simulink model "Six_Step_Commutation"  (R2022b)
settings: Solver=FixedStepAuto  StartTime=0.0  StopTime=inf  FixedStep=50e-6  RelTol=1e-3
undefined symbols (not defined in the file): IO397, pull, up
libraries: speedgoatlib_fpga_pwm x1, speedgoatlib_fpga_dio x1, simulink x1, speedgoatlib_fpga x1
settings Model: SimulationMode=external  ExtModeEnableFloating=off  ExtModeTrigDuration=100000  Creator=safder.1  LastModifiedBy=safder.1
settings SolverCC: ConcurrentTasks=on  PositivePriorityOrder=on  AutoInsertRateTranBlk=on
settings OptimizationCC: BlockReduction=off  OptimizeBlockIOStorage=off
settings DebuggingCC: TasksWithSamePriorityMsg=none
settings HardwareCC: ProdBitPerLong=64  ProdLongLongMode=on  ProdHWDeviceType=Intel->x86-64 (Linux 64)
settings RTWCC: Description=Simulink Real-Time  SystemTargetFile=slrealtime.tlc  TemplateMakefile=slrealtime_default_tmf  Toolchain=Simulink Real-Time Toolchain  BuildConfiguration=Faster Runs  CodeExecutionProfiling=on  TargetLang=C++

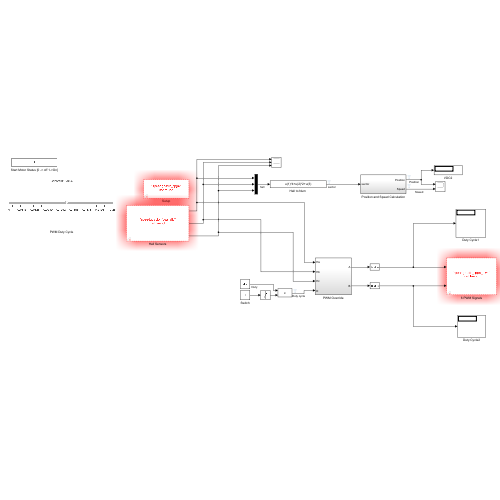
[thumbnail: Simulink's stored preview of the top-level diagram]
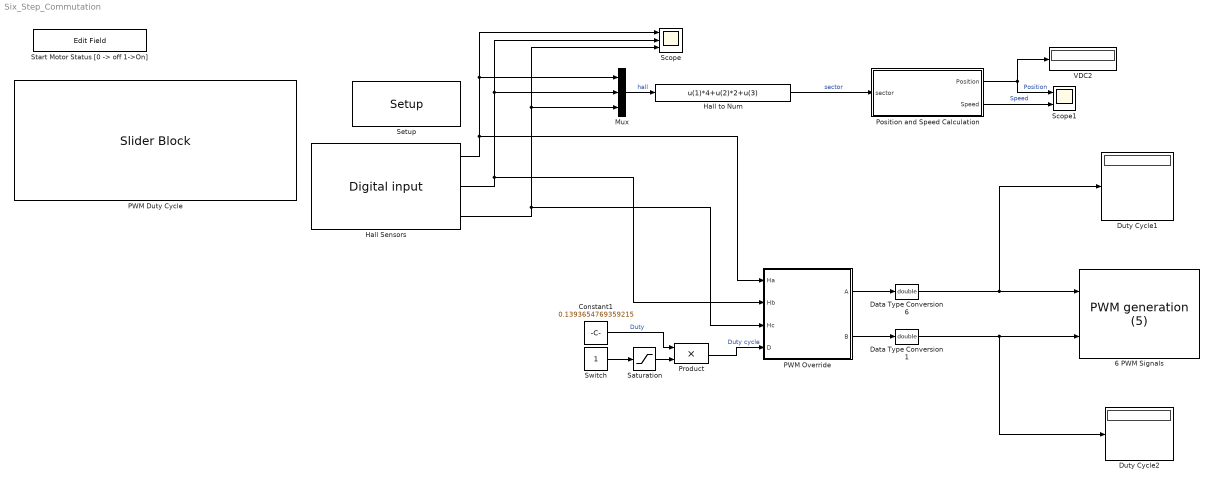
== system Six_Step_Commutation ==
  6 PWM Signals : speedgoatlib_fpga_pwm/PWM generation (5)  id=1  chan=[1 2 3]  board=Please select...  ts=0.0001  enableDma=off  pciSlot=-1  delay=0  symmetric=Symmetric - PWM generation is centered around half the period  b_is_complement_of_a=Independent of PWM A output  deadband=[0.0000025]  period=0.0001  frequency=10000  ticks=7499  a_on=[0]  a_off=[0]  pwm_a_dc=[0.0]  b_on=[0]  b_off=[0]  pwm_b_dc=[0]  c_on=[0.0]  c_off=[0.0]  protection=Disabled: A and B can be high at the same moment  enable_latch_half_period=off  pwm_update=At period starts  bit_width_pwm_gen=24  trigger_duration=[1e-6]  trigger_period_start=off  trigger_half_of_the_period=off  trigger_a_on=off  trigger_a_off=off  trigger_b_on=off  trigger_b_off=off  show_a_input=on  show_b_input=on  show_c_input=off  show_period_input=off  show_force_stop_input=off  idle_a=Low when PWM generation is halted  idle_b=Low when PWM generation is halted  idle_c=Low when PWM generation is halted  cancels_pwm_generation=on  invert_a=off  invert_b=off  invert_c=off
  Constant1 : Constant  Value=0.1393654769359215
  Data Type Conversion1 : DataTypeConversion  OutDataTypeStr=double  SaturateOnIntegerOverflow=off  RndMeth=Floor
  Data Type Conversion6 : DataTypeConversion  OutDataTypeStr=double  SaturateOnIntegerOverflow=off  RndMeth=Floor
  Duty Cycle1 : Display
  Duty Cycle2 : Display
  Hall Sensors : speedgoatlib_fpga_dio/Digital input  id=1  chan=[11 12 13]  ts=0.0001  vectorizeOutput=off
  "Hall to Num " : Fcn  Expr=u(1)*4+u(2)*2+u(3)
  Mux : Mux  Inputs=3
  PWM Duty Cycle : SliderBlock  ScaleMax=0.25
  PWM Override : Subsystem
  Position and Speed Calculation : Subsystem
  Product : Product
  Saturation : Saturate  UpperLimit=1  LowerLimit=0
  Scope : Scope  NumInputPorts=3
  Scope1 : Scope  NumInputPorts=2
  Setup : speedgoatlib_fpga/Setup/Setup  Parameter124={}  board=IO397-50k  id=1  pciSlot=-1  device_id=1  bitstreamFilePath=C:\ProgramData\Speedgoat\bitstreams\io_configuration_package\R2022b\io397  bitstreamFile=speedgoat_IO397_RCP.mat  rearEnb_1=off  rearIO_1=None  rearEnb_2=off  rearIO_2=None  ProgSpiFlash=off  ProgBPIFlash=off  useFpgaDmaController=off  PullRPort15=pull-up 3.3V  PullRPort31=pull-up 3.3V  PullRPort47=pull-up 3.3V  PullRPort63=pull-up 3.3V  diffLineTermination_1=on  diffLineTermination_2=on  diffLineTermination_3=on  diffLineTermination_4=on  diffLineTermination_5=on  diffLineTermination_6=on  diffLineTermination_7=on  diffLineTermination_8=on  diffLineTermination_9=on  diffLineTermination_10=on  diffLineTermination_11=on  diffLineTermination_12=on  diffLineTermination_13=on  diffLineTermination_14=on  diffLineTermination_15=on  diffLineTermination_16=on  diffLineTermination_17=on  diffLineTermination_18=on  diffLineTermination_19=on  diffLineTermination_20=on  diffLineTermination_21=on  diffLineTermination_22=on  diffLineTermination_23=on  diffLineTermination_24=on  diffLineTermination_25=on  diffLineTermination_26=on  diffLineTermination_27=on  diffLineTermination_28=on  diffLineTermination_29=on  diffLineTermination_30=on  diffLineTermination_31=on  diffLineTermination_32=on  Vi_Pull_36x_1=Floating  Vo_36x_1=3.3V  Vi_Pull_36x_2=Floating  Vo_36x_2=3.3V  Vi_Pull_36x_3=Floating  Vo_36x_3=3.3V  Vi_Pull_36x_4=Floating  Vo_36x_4=3.3V  Vi_Pull_36x_5=Floating  Vo_36x_5=3.3V  Vi_Pull_36x_6=Floating  Vo_36x_6=3.3V  Vi_Pull_36x_7=Floating  Vo_36x_7=3.3V  Vi_Pull_36x_8=Floating  Vo_36x_8=3.3V  Vi_Pull_36x_9_16=Floating  Vo_36x_9_16=3.3V  Vi_Pull_36x_17_24=Floating  Vo_36x_17_24=3.3V  Vi_Pull_36x_25_32=Floating  Vo_36x_25_32=3.3V  Vi_Pull_36x_33_40=Floating  Vo_36x_33_40=3.3V  Vi_Pull_36x_41_48=Floating  Vo_36x_41_48=3.3V  Vi_Pull_36x_49_56=Floating  Vo_36x_49_56=3.3V  Vi_Pull_36x_57_64=Floating  Vo_36x_57_64=3.3V  PullRPort0_1=pull-up  VioPort0_1=3.3V  PullRPort1_1=pull-up  VioPort1_1=3.3V  PullRPort2_1=pull-up  VioPort2_1=3.3V  PullRPort3_1=pull-up  VioPort3_1=3.3V  PullRPort4_1=pull-up  VioPort4_1=3.3V  PullRPort5_1=pull-up  VioPort5_1=3.3V  PullRPort6_1=pull-up  VioPort6_1=3.3V  diffLineTermination_rear1_1=on  diffLineTermination_rear1_2=on  diffLineTermination_rear1_3=on  diffLineTermination_rear1_4=on  diffLineTermination_rear1_5=on  diffLineTermination_rear1_6=on  diffLineTermination_rear1_7=on  diffLineTermination_rear1_8=on  PullRPort0_2=pull-up  VioPort0_2=3.3V  PullRPort1_2=pull-up  VioPort1_2=3.3V  PullRPort2_2=pull-up  VioPort2_2=3.3V  PullRPort3_2=pull-up  VioPort3_2=3.3V  PullRPort4_2=pull-up  VioPort4_2=3.3V  PullRPort5_2=pull-up  VioPort5_2=3.3V  PullRPort6_2=pull-up  VioPort6_2=3.3V  diffLineTermination_rear2_1=on  diffLineTermination_rear2_2=on  diffLineTermination_rear2_3=on  diffLineTermination_rear2_4=on  diffLineTermination_rear2_5=on  diffLineTermination_rear2_6=on  diffLineTermination_rear2_7=on  diffLineTermination_rear2_8=on
  "Start Motor Status [0 -> off 1->On]" : EditField  LabelPosition=Hide  ShowInitialText=on  Alignment=Center
  Switch : Constant
  VDC2 : Display
  wires:
  Mux/1 -> "Hall to Num "/1  "hall"
  Hall Sensors/1 -> PWM Override/1(Ha), Scope/1, Mux/1
  Hall Sensors/2 -> Mux/2, Scope/2, PWM Override/2(Hb)
  Hall Sensors/3 -> PWM Override/3(Hc), Scope/3, Mux/3
  PWM Override/1(A) -> Data Type Conversion6/1
  PWM Override/2(B) -> Data Type Conversion1/1
  Data Type Conversion6/1 -> 6 PWM Signals/1, Duty Cycle1/1
  Data Type Conversion1/1 -> 6 PWM Signals/2, Duty Cycle2/1
  "Hall to Num "/1 -> Position and Speed Calculation/1(sector)  "sector"
  Position and Speed Calculation/2(Speed) -> Scope1/2  "Speed"
  Position and Speed Calculation/1(Position) -> VDC2/1, Scope1/1  "Position"
  Switch/1 -> Saturation/1
  Saturation/1 -> Product/2
  Constant1/1 -> Product/1  "Duty"
  Product/1 -> PWM Override/4(D)  "Duty cycle"

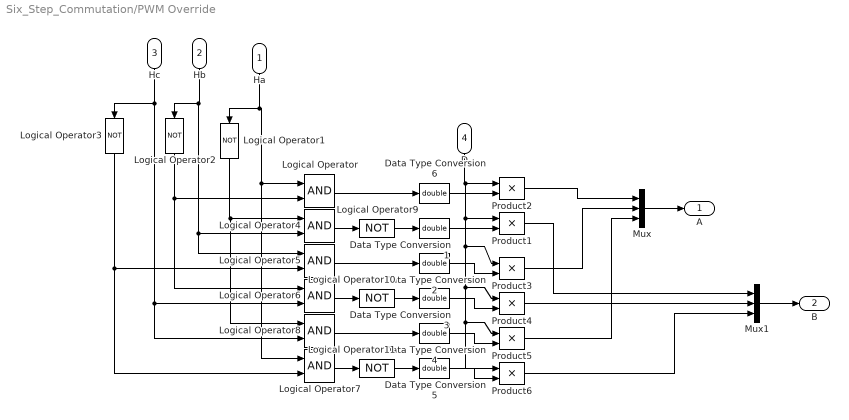
== system Six_Step_Commutation/PWM Override ==
  Ha : Inport
  Hb : Inport  Port=2
  Hc : Inport  Port=3
  D : Inport  Port=4
  Data Type Conversion{1..6} (6 alike) : DataTypeConversion  OutDataTypeStr=double  SaturateOnIntegerOverflow=off  RndMeth=Floor
  Logical Operator{,4..8} (6 alike) : Logic  AllPortsSameDT=off  OutDataTypeStr=boolean
  Logical Operator{1..3,9..11} (6 alike) : Logic  Operator=NOT  AllPortsSameDT=off  OutDataTypeStr=boolean
  Mux : Mux  Inputs=3
  Mux1 : Mux  Inputs=3
  Product{1..6} (6 alike) : Product
  A : Outport
  B : Outport  Port=2
  wires:
  Hc/1 -> Logical Operator8/2, Logical Operator6/2, Logical Operator3/1
  Hb/1 -> Logical Operator5/1, Logical Operator4/2, Logical Operator2/1
  Ha/1 -> Logical Operator7/1, Logical Operator/1, Logical Operator1/1
  Logical Operator4/1 -> Logical Operator9/1
  Data Type Conversion6/1 -> Product2/2
  Data Type Conversion1/1 -> Product1/2
  Data Type Conversion2/1 -> Product3/2
  Data Type Conversion3/1 -> Product4/2
  Data Type Conversion4/1 -> Product5/2
  Data Type Conversion5/1 -> Product6/2
  Logical Operator/1 -> Data Type Conversion6/1
  Product2/1 -> Mux/1
  Product3/1 -> Mux/2
  Product5/1 -> Mux/3
  Product1/1 -> Mux1/1
  Product4/1 -> Mux1/2
  Product6/1 -> Mux1/3
  D/1 -> Product2/1, Product1/1, Product3/1, Product4/1, Product5/1, Product6/1
  Logical Operator5/1 -> Data Type Conversion2/1
  Logical Operator6/1 -> Logical Operator10/1
  Logical Operator8/1 -> Data Type Conversion4/1
  Logical Operator7/1 -> Logical Operator11/1
  Logical Operator2/1 -> Logical Operator6/1, Logical Operator/2
  Logical Operator1/1 -> Logical Operator8/1, Logical Operator4/1
  Logical Operator3/1 -> Logical Operator7/2, Logical Operator5/2
  Logical Operator9/1 -> Data Type Conversion1/1
  Logical Operator10/1 -> Data Type Conversion3/1
  Logical Operator11/1 -> Data Type Conversion5/1
  Mux/1 -> A/1
  Mux1/1 -> B/1

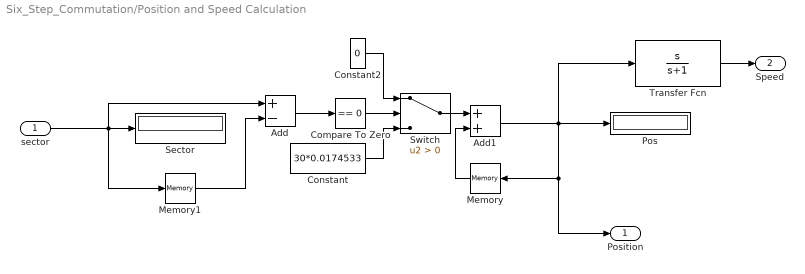
== system Six_Step_Commutation/Position and Speed Calculation ==
  sector : Inport
  Add : Sum  Inputs=+-
  Add1 : Sum
  Compare To Zero : simulink/Logic and Bit Operations/Compare To Zero  relop===  OutDataTypeStr=boolean
  Constant : Constant  Value=30*0.0174533  SampleTime=0.001
  Constant2 : Constant  Value=0  SampleTime=0.001
  Memory : Memory
  Memory1 : Memory
  Pos : Display
  Sector : Display
  Switch : Switch  Criteria=u2 > Threshold  SaturateOnIntegerOverflow=off  InputSameDT=off
  Transfer Fcn : TransferFcn  Numerator=[1 0]  Denominator=[1 1]
  Position : Outport
  Speed : Outport  Port=2
  wires:
  sector/1 -> Memory1/1, Add/1, Sector/1
  Compare To Zero/1 -> Switch/2
  Constant/1 -> Switch/3
  Add/1 -> Compare To Zero/1
  Constant2/1 -> Switch/1
  Transfer Fcn/1 -> Speed/1
  Switch/1 -> Add1/1
  Add1/1 -> Transfer Fcn/1, Memory/1, Position/1, Pos/1
  Memory/1 -> Add1/2
  Memory1/1 -> Add/2
